simulink model "C172S_PitchAttitudeHold_V1"  (R2026a)
settings: Solver=ode4  StartTime=0  StopTime=60  FixedStep=0.01
InitFcn:
  | paData = c172sLongitudinalData();
  | [~, paPlant] = c172sLongitudinalPlant(paData);
  | paDamper = c172sPitchRateDamperData();
  | paController = c172sPitchAttitudeControllerData();
  | A_pa = paPlant.A; B_pa = paPlant.B;
  | C_pa = paPlant.C; D_pa = paPlant.D;
  | Kq_pa_s = paDamper.Kq_s;
  | Kp_pa = paController.Kp_radPerRad;
  | Ki_pa_per_s = paController.Ki_radPerRadPerS;
  | tauThetaCommand_pa_s = paController.commandFilterTimeConstant_s;
  | thetaCommandStep_pa_rad = deg2rad(paController.validation.commandStep_deg);
  | deltaEBias_pa_rad = 0.0;
  | x0_pa = zeros(4,1); xi0_pa = 0.0;
settings Model: Creator=Shahi  LastModifiedBy=Shahi

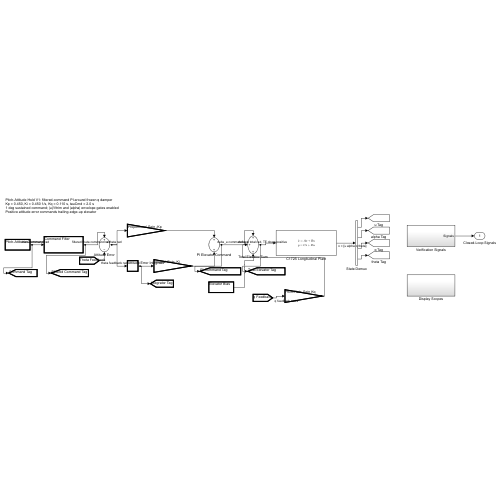
[thumbnail: Simulink's stored preview of the top-level diagram]
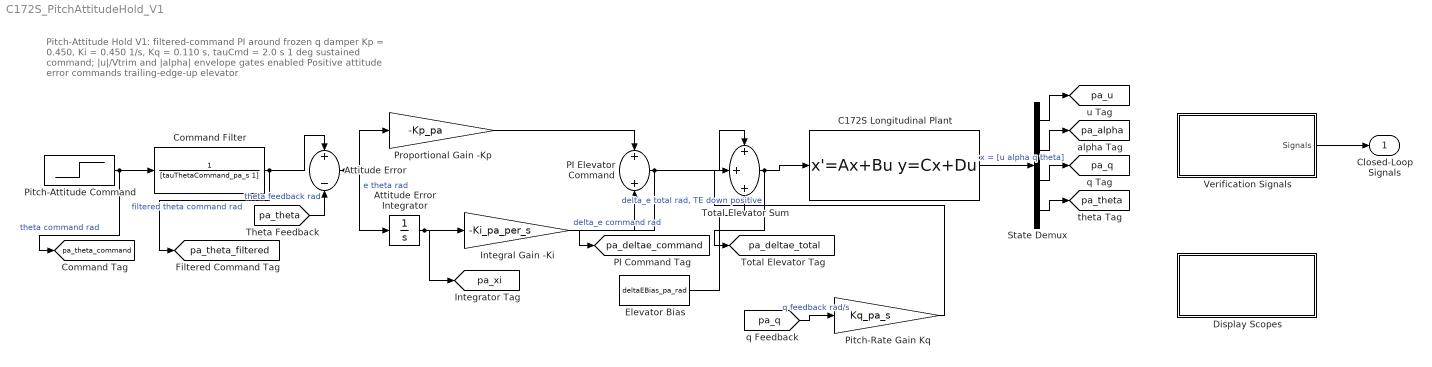
== system C172S_PitchAttitudeHold_V1 ==
  note: Pitch-Attitude Hold V1: filtered-command PI around frozen q damper
      | Kp = 0.450, Ki = 0.450 1/s, Kq = 0.110 s, tauCmd = 2.0 s
      | 1 deg sustained command; |u|/Vtrim and |alpha| envelope gates enabled
      | Positive attitude error commands trailing-edge-up elevator
  Attitude Error : Sum  Inputs=+-
  Attitude Error Integrator : Integrator  InitialCondition=xi0_pa
  C172S Longitudinal Plant : StateSpace  A=A_pa  B=B_pa  C=C_pa  D=D_pa  InitialCondition=x0_pa
  Command Filter : TransferFcn  Numerator=1  Denominator=[tauThetaCommand_pa_s 1]
  Display Scopes : Subsystem
  Elevator Bias : Constant  Value=deltaEBias_pa_rad  SampleTime=0
  Integral Gain -Ki : Gain  Gain=-Ki_pa_per_s
  PI Elevator Command : Sum
  Pitch-Attitude Command : Step  Time=0.0  InitialValue=0.0  FinalValue=thetaCommandStep_pa_rad  SampleTime=0
  Pitch-Rate Gain Kq : Gain  Gain=Kq_pa_s
  Proportional Gain -Kp : Gain  Gain=-Kp_pa
  State Demux : Demux
  Total Elevator Sum : Sum  Inputs=+++
  Verification Signals : Subsystem
  Closed-Loop Signals : Outport
  tag scope: pa_alpha=global, pa_deltae_command=global, pa_deltae_total=global, pa_q=global, pa_theta=global, pa_theta_command=global, pa_theta_filtered=global, pa_u=global, pa_xi=global
  wires:
  Verification Signals/1(Signals) -> Closed-Loop Signals/1
  Pitch-Attitude Command/1 -> Command Filter/1, [pa_theta_command]  "theta command rad"
  Command Filter/1 -> Attitude Error/1, [pa_theta_filtered]  "filtered theta command rad"
  Attitude Error/1 -> Proportional Gain -Kp/1, Attitude Error Integrator/1  "e theta rad"
  Proportional Gain -Kp/1 -> PI Elevator Command/1
  Attitude Error Integrator/1 -> Integral Gain -Ki/1, [pa_xi]
  Integral Gain -Ki/1 -> PI Elevator Command/2
  PI Elevator Command/1 -> Total Elevator Sum/1, [pa_deltae_command]  "delta_e command rad"
  Pitch-Rate Gain Kq/1 -> Total Elevator Sum/2
  Elevator Bias/1 -> Total Elevator Sum/3
  Total Elevator Sum/1 -> C172S Longitudinal Plant/1, [pa_deltae_total]  "delta_e total rad, TE down positive"
  C172S Longitudinal Plant/1 -> State Demux/1  "x = [u alpha q theta]"
  [pa_theta] -> Attitude Error/2  "theta feedback rad"
  [pa_q] -> Pitch-Rate Gain Kq/1  "q feedback rad/s"
  State Demux/1 -> [pa_u]
  State Demux/2 -> [pa_alpha]
  State Demux/3 -> [pa_q]
  State Demux/4 -> [pa_theta]

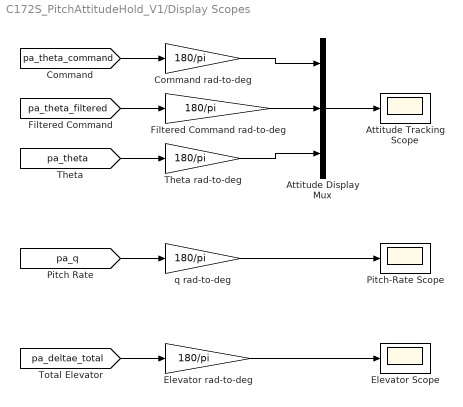
== system C172S_PitchAttitudeHold_V1/Display Scopes ==
  Attitude Display Mux : Mux  Inputs=3
  Attitude Tracking Scope : Scope
  Command rad-to-deg : Gain  Gain=180/pi
  Elevator Scope : Scope
  Elevator rad-to-deg : Gain  Gain=180/pi
  Filtered Command rad-to-deg : Gain  Gain=180/pi
  Pitch-Rate Scope : Scope
  Theta rad-to-deg : Gain  Gain=180/pi
  q rad-to-deg : Gain  Gain=180/pi
  wires:
  [pa_theta_command] -> Command rad-to-deg/1
  Command rad-to-deg/1 -> Attitude Display Mux/1
  [pa_theta_filtered] -> Filtered Command rad-to-deg/1
  Filtered Command rad-to-deg/1 -> Attitude Display Mux/2
  [pa_theta] -> Theta rad-to-deg/1
  Theta rad-to-deg/1 -> Attitude Display Mux/3
  Attitude Display Mux/1 -> Attitude Tracking Scope/1
  [pa_q] -> q rad-to-deg/1
  q rad-to-deg/1 -> Pitch-Rate Scope/1
  [pa_deltae_total] -> Elevator rad-to-deg/1
  Elevator rad-to-deg/1 -> Elevator Scope/1

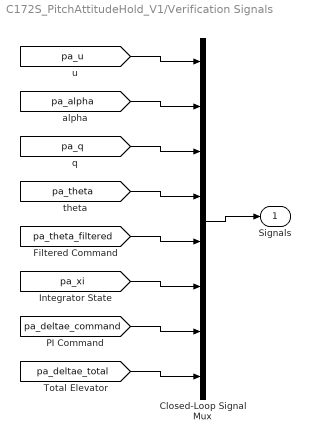
== system C172S_PitchAttitudeHold_V1/Verification Signals ==
  Closed-Loop Signal Mux : Mux  Inputs=8
  Signals : Outport
  wires:
  [pa_u] -> Closed-Loop Signal Mux/1
  [pa_alpha] -> Closed-Loop Signal Mux/2
  [pa_q] -> Closed-Loop Signal Mux/3
  [pa_theta] -> Closed-Loop Signal Mux/4
  [pa_theta_filtered] -> Closed-Loop Signal Mux/5
  [pa_xi] -> Closed-Loop Signal Mux/6
  [pa_deltae_command] -> Closed-Loop Signal Mux/7
  [pa_deltae_total] -> Closed-Loop Signal Mux/8
  Closed-Loop Signal Mux/1 -> Signals/1
